simulink model "lab2_przyklad2"  (R2021b)
settings: Solver=VariableStepAuto  StartTime=0.0  StopTime=20  RelTol=1e-3  EnableMultiTasking=on
settings Model: Creator=dsych  LastModifiedBy=dsych
settings SolverCC: AlgebraicLoopSolver=TrustRegion
settings DataIOCC: ReturnWorkspaceOutputs=off
settings OptimizationCC: LifeSpan=inf
settings DebuggingCC: SFUnexpectedBacktrackingDiag=warning  SFNoUnconditionalDefaultTransitionDiag=warning  SFMachineParentedDataDiag=warning  ArithmeticOperatorsInVariantConditions=warning
settings SFSimCC: SimUseLocalCustomCode=off  CustomCodeUndefinedFunction=UseInterfaceOnly
settings RTWCC: RTWUseLocalCustomCode=off
settings CodeAppCC: StateflowObjectComments=on
settings GRTTargetCC: TargetLangStandard=C89/C90 (ANSI)
settings ConfigComp: CovMetricSettings=dw  CovSaveCumulativeToWorkspaceVar=on  CovSaveSingleToWorkspaceVar=on  CovExternalEMLEnable=off

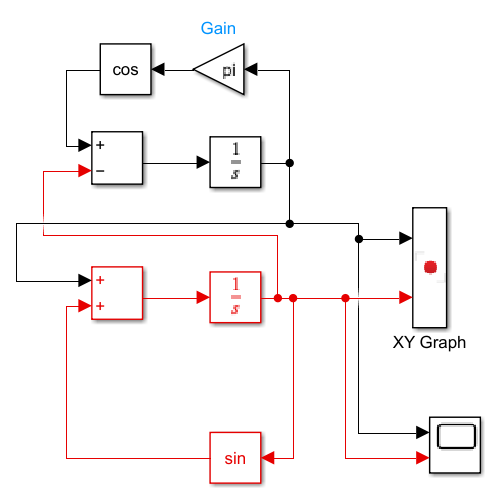
[thumbnail: Simulink's stored preview of the top-level diagram]
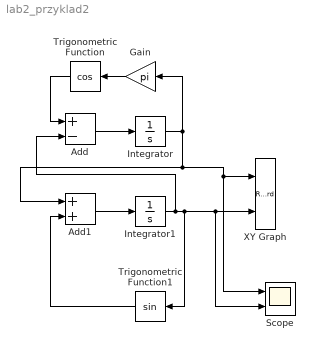
== system lab2_przyklad2 ==
  Add : Sum  Inputs=+-
  Add1 : Sum
  Gain : Gain  Gain=pi
  Integrator : Integrator  InitialCondition=70
  Integrator1 : Integrator  InitialCondition=1
  Scope : Scope  NumInputPorts=2
  Trigonometric Function : Trigonometry  Operator=cos
  Trigonometric Function1 : Trigonometry
  XY Graph : Record  FileSettingsInternal="{\"entries\":[{\"content\":{\"excelSettings\":{\"content\":{},\"type\":\"Streamout.ExcelSettings\"}},\"type\":\"Streamout.FileSettingStorage\",\"uuid\":\"3123b390-ef3e-4de2-a824-38e625c7bc38\"}],\"packageUris\":[\"http://schema.mathworks.com/mf0/streamout_blocks/R2020a\"],\"version\":\"1.0\"}"  Layout=[1 1]  SignalsInternal="{\"entries\":[{\"content\":{\"signals\":[{\"content\":{\"blockPath\":[\"lab2_przyklad2/XY Graph\"],\"channel\":[],\"dimensions\":[1],\"domain\":\"lab2_przyklad2/XY Graph\",\"lineColor\":\"#a2142f\",\"plots\":[1],\"port\":1,\"sid\":[\"\"],\"signalID\":180,\"signalName\":\"Integrator\"},\"type\":\"RecordBlkView.Signal\",\"uuid\":\"ca65626a-e239-4f48-a58e-dbfef03081ce\"},{\"content\":{\"blockPath\":[\"lab2_przyklad2/XY Graph\"],\"channel\":[],\"dimensions\":[1],\"domain\":\"lab2_przyklad2/XY Graph\",\"lineColor\":\"#139fff\",\"plots\":[1],\"port\":2,\"sid\":[\"\"],\"signalID\":184,\"signalName\":\"Integrator1\"},\"type\":\"RecordBlkView.Signal\",\"uuid\":\"9d33eba4-f19b-4dfa-9d83-e978483bcace\"}]},\"type\":\"RecordBlkView.InputSignals\",\"uuid\":\"65e2a600-c13a-4bf2-9abb-be18f638527b\"}],\"packageUris\":[\"http://schema.mathworks.com/mf0/streamout_blocks/R2020a\"],\"version\":\"1.0\"}"  VisualizationBindings="{\"xyplotplugin\":{\"info\":[{\"series\":[{\"bindingParametersList\":[{\"parameter\":\"X-Axis\",\"signalID\":180,\"signalName\":\"Integrator\"},{\"parameter\":\"Y-Axis\",\"signalID\":184,\"signalName\":\"Integrator1\"}],\"seriesID\":11445}],\"subplotID\":1}]}}"  CompatibilityTag=XY  st=-1
  wires:
  Add/1 -> Integrator/1
  Add1/1 -> Integrator1/1
  Gain/1 -> Trigonometric Function/1
  Trigonometric Function/1 -> Add/1
  Integrator1/1 -> Add/2, XY Graph/2, Scope/2, Trigonometric Function1/1
  Integrator/1 -> Scope/1, XY Graph/1, Add1/1, Gain/1
  Trigonometric Function1/1 -> Add1/2
